simulink model "Option_3"  (R2023b)
settings: Solver=VariableStepAuto  StartTime=0.0  StopTime=25  RelTol=1e-3
values from neighbouring files (symbols this model uses):
  A_current = current_values.(4)    [Part1.m]    (also in Part2.m = A(x))
  b1 = 1    [Part2.m]
  b2 = 1    [Part2.m]
  J1 = 100    [Part2.m]
settings Model: Creator=jessi  LastModifiedBy=jessi

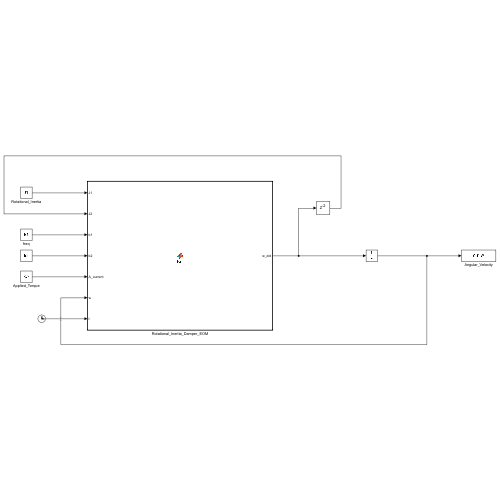
[thumbnail: Simulink's stored preview of the top-level diagram]
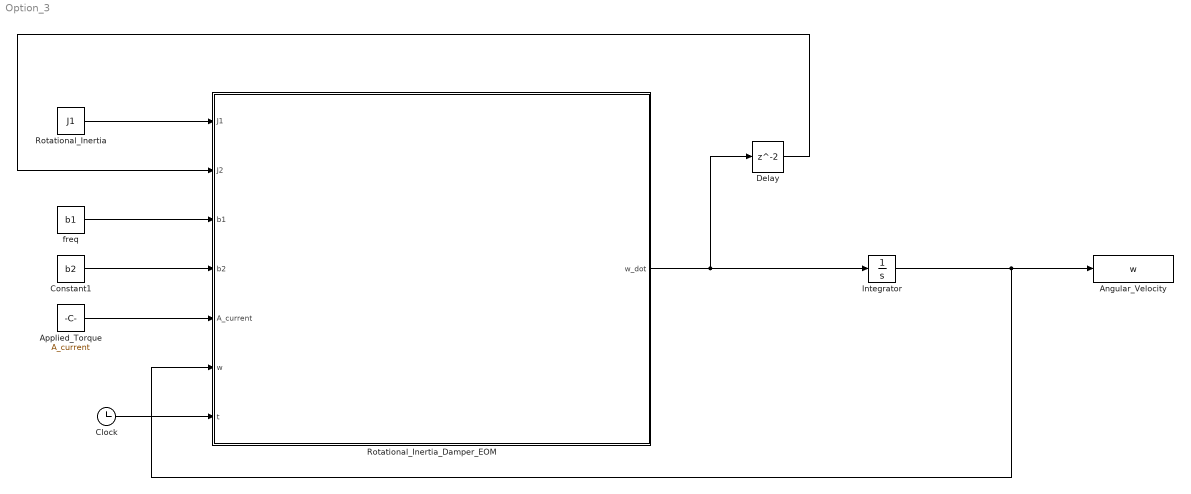
== system Option_3 ==
  Angular_Velocity : ToWorkspace  VariableName=w  SaveFormat=Timeseries  SampleTime=-1
  Applied_Torque : Constant  Value=A_current
  Clock : Clock
  Constant1 : Constant  Value=b2
  Delay : Delay
  Integrator : Integrator
  Rotational_Inertia : Constant  Value=J1
  Rotational_Inertia_Damper_EOM : MATLAB Function  TreatAsAtomicUnit=on
  freq : Constant  Value=b1
  wires:
  Integrator/1 -> Rotational_Inertia_Damper_EOM/6(w), Angular_Velocity/1
  Rotational_Inertia_Damper_EOM/1(w_dot) -> Delay/1, Integrator/1
  freq/1 -> Rotational_Inertia_Damper_EOM/3(b1)
  Constant1/1 -> Rotational_Inertia_Damper_EOM/4(b2)
  Clock/1 -> Rotational_Inertia_Damper_EOM/7(t)
  Applied_Torque/1 -> Rotational_Inertia_Damper_EOM/5(A_current)
  Rotational_Inertia/1 -> Rotational_Inertia_Damper_EOM/1(J1)
  Delay/1 -> Rotational_Inertia_Damper_EOM/2(J2)

== matlab function Option_3/Rotational_Inertia_Damper_EOM ==
  data: J1 input; w_dot output; J2 input; b1 input; b2 input; A_current input; w input; t input
function w_dot = fcn(J1,J2,b1,b2,A_current,w,t)

w_dot = (1/(J1+J2))*(A_current-(b1+b2)*w);
J2 = J1;

end
